simulink model "StateSpaceSim"  (R2017a)
settings: Solver=VariableStepAuto  StartTime=0.0  StopTime=10.0  RelTol=1e-3
values from neighbouring files (symbols this model uses):
  A = [ -1*M0(TermR)/M0(TermL) 0 0 0 -1*M0(SpdK)/M0(TermL) 0 0 0 ... (first row only)    [StateSpace.m]
  B = [1 0 0 0 ... (first row only)    [StateSpace.m]
  C = 2*linearizedThrustGain*RadSec_SS*DroneMomentArm*[0 0 0 0 1 -1 0 0 ... (first row only)    [StateSpace.m]
  D = zeros(2,4)    [StateSpace.m]
settings Model: Creator=Matthew  LastModifiedBy=Matthew

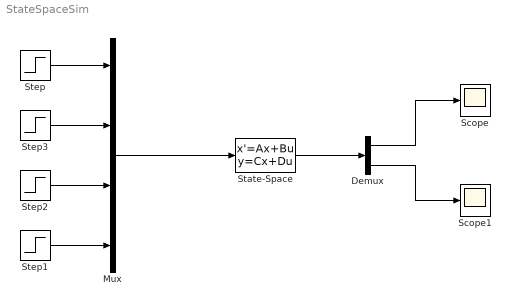
== system StateSpaceSim ==
  Demux : Demux  Outputs=2
  Mux : Mux
  Scope : Scope
  Scope1 : Scope
  State-Space : StateSpace  A=A  B=B  C=C  D=D  X0=0
  Step{,1..3} (4 alike) : Step  SampleTime=0
  wires:
  Step/1 -> Mux/1
  Step3/1 -> Mux/2
  Step2/1 -> Mux/3
  Step1/1 -> Mux/4
  Mux/1 -> State-Space/1
  State-Space/1 -> Demux/1
  Demux/1 -> Scope/1
  Demux/2 -> Scope1/1
